simulink model "Q8"  (R2023a)
settings: Solver=VariableStepAuto  StartTime=0.0  StopTime=3  RelTol=1e-3
libraries: spsControlledVoltageSourceLib x3, spsAsynchronousMachineSIUnitsLib x1, spsGroundLib x1, eeProgrammableSignalGenerator x1, spspowerguiLib x1
settings Model: Creator=mango  LastModifiedBy=eij22jb
settings OptimizationCC: ReuseModelBlockBuffer=off

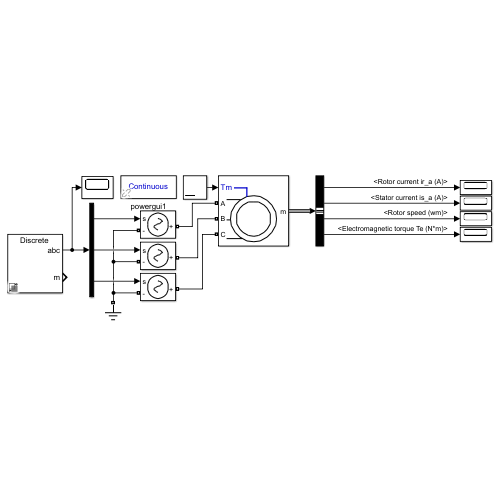
[thumbnail: Simulink's stored preview of the top-level diagram]
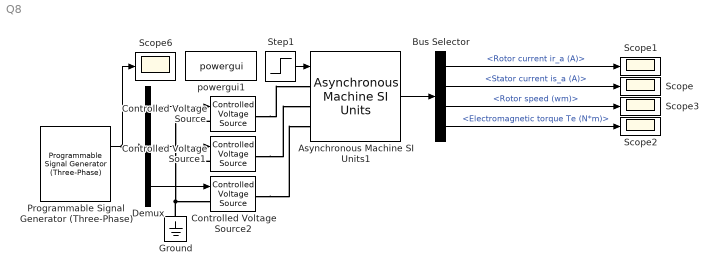
== system Q8 ==
  Asynchronous Machine SI Units1 : spsAsynchronousMachineSIUnitsLib/Asynchronous Machine SI Units  RotorType=Squirrel-cage  PresetModel=No  MechanicalLoad=Torque Tm  ShowDetailedParameters=on  ReferenceFrame=Rotor  Units=SI  MeasurementBus=off  NominalParameters=[9325 400 50]  VoltageRatio=1  Stator=[0.8 0.00907]  Rotor=[0.8 0.00907]  Cage1=[0.4155 0.002066]  Cage2=[0.4168 0.0003495]  Lm=0.637  Mechanical=[0.1 0 2]  PolePairs=2  InitialConditions=[1 0 0 0 0 0 0 0]  SimulateSaturation=off  Saturation=[14.03593122, 27.81365428, 53.79336849, 72.68890987, 97.98006896, 148.6815601, 215.7428561, 302.9841135, 428.7778367 ; 230, 322, 414, 460, 506, 552, 598, 644, 690]  LoadFlowParameters=1492000  TsPowergui=0  TsBlock=-1  IterativeModel=Trapezoidal non iterative  IterativeDiscreteModel=Trapezoidal non iterative  Pmec=1.492e+006
  Bus Selector : BusSelector  OutputSignals=Rotor measurements.Rotor current ir_a (A),Stator measurements.Stator current is_a (A),Mechanical.Rotor speed (wm),Mechanical.Electromagnetic torque Te (N*m)
  Controlled Voltage Source : spsControlledVoltageSourceLib/Controlled Voltage Source  Initialize=on  Source_Type=AC  Amplitude=0  Phase=0  Frequency=0  Measurements=None
  Controlled Voltage Source1 : spsControlledVoltageSourceLib/Controlled Voltage Source  Initialize=on  Source_Type=AC  Amplitude=0  Phase=-120  Frequency=0  Measurements=None
  Controlled Voltage Source2 : spsControlledVoltageSourceLib/Controlled Voltage Source  Initialize=on  Source_Type=AC  Amplitude=0  Phase=0  Frequency=0  Measurements=None
  Demux : Demux  Outputs=3
  Ground : spsGroundLib/Ground  LConnTagsString=a
  Programmable Signal Generator (Three-Phase) : eeProgrammableSignalGenerator/Programmable Signal Generator (Three-Phase)  LabelModeActiveChoice=Discrete  VariationAmplitude=Ramp  Amp=0  Amp_RampRate=230*sqrt(2)/0.5  Amp_StepValue=100  Amp_ModulationMag=50  Amp_ModulationFreq=10  Amp_Tstart=0  Amp_Tstop=0.5  Amp_Table=[0 30 60 90]  Amp_Time=[0 0.3 0.6 0.9]  VariationFrequency=Ramp  Freq=5  Freq_RampRate=45/0.5  Freq_StepValue=100  Freq_ModulationMag=50  Freq_ModulationFreq=10  Freq_Tstart=0  Freq_Tstop=0.5  Freq_Table=[0 30 60 90]  Freq_Time=[0 0.3 0.6 0.9]  VariationPhase=Constant  Phase=0  Phase_RampRate=100  Phase_StepValue=100  Phase_ModulationMag=50  Phase_ModulationFreq=10  Phase_Tstart=0.1  Phase_Tstop=0.6  Phase_Table=[0 30 60 90]  Phase_Time=[0 0.3 0.6 0.9]  Harmo_En1=off  Harmo_Seq1=Zero Sequence  Harmo_Ord1=3  Harmo_Mag1=50  Harmo_Phase1=180  Harmo_Tstart1=0.1  Harmo_Tstop1=0.6  Harmo_En2=off  Harmo_Seq2=Zero Sequence  Harmo_Ord2=3  Harmo_Mag2=50  Harmo_Phase2=180  Harmo_Tstart2=0.1  Harmo_Tstop2=0.6  Ts=1e-4
      settings: LibrarySourceBlock=|
      | ee_sl_lib/General Control/Programmable
      | Signal Generator (Three-Phase)
  Scope{,1..3,6} (5 alike) : Scope
  Step1 : Step  Time=1.5  After=49.89  SampleTime=0
  powergui1 : spspowerguiLib/powergui  Priority=1  SimulationMode=Continuous  SampleTime=50e-6  frequency=60  Iterations=50  frequencyindice=50  Pbase=100e6  ErrMax=1e-4  UnitsV=kV  UnitsW=MW  buscounter=0  FunctionMessages=off  echomessages=off  EnableUseOfTLC=off  CurrentSourceSwitches=off  DisableSnubberDevices=off  DisableRonSwitches=off  DisableVfSwitches=off  DisplayEquations=off  AutomaticDiscreteSolvers=off  SolverType=Tustin/Backward Euler (TBE)  Interpol=off  ExternalGateDelay=off  methode=off  Ts=100  x0status=blocks  SPID=on  SwTol=0  HookPort=off  NonlinearTolerance=1e-4  nMaxIteration=100  ContinueOnMaxIteration=off  RestoreLinks=warning  ResistiveCurrentMeasurement=off  Frange=[0:2:500]  Ylog=off  Xlog=on  ShowGrid=off  save=off  variable=ZData  structure=0  ZoomFFT=off  StartTime=0.0  cycles=1  DisplayStyle=1  fundamental=60  FreqAxis=off  MaxFrequency=1000  frequencyindicesteady=1  RmsSteady=1  display=off
  wires:
  Asynchronous Machine SI Units1/1 -> Bus Selector/1
  Bus Selector/3 -> Scope3/1  "<Rotor speed (wm)>"
  Bus Selector/1 -> Scope1/1  "<Rotor current ir_a (A)>"
  Bus Selector/2 -> Scope/1  "<Stator current is_a (A)>"
  Bus Selector/4 -> Scope2/1  "<Electromagnetic torque Te (N*m)>"
  Step1/1 -> Asynchronous Machine SI Units1/1
  Demux/1 -> Controlled Voltage Source/1
  Demux/2 -> Controlled Voltage Source1/1
  Demux/3 -> Controlled Voltage Source2/1
  Programmable Signal Generator (Three-Phase)/1 -> Scope6/1, Demux/1
  connections:
  Ground/LConn1 -- Controlled Voltage Source/LConn1 -- Controlled Voltage Source1/LConn1 -- Controlled Voltage Source2/LConn1
  Controlled Voltage Source/RConn1 -- Asynchronous Machine SI Units1/LConn1
  Controlled Voltage Source1/RConn1 -- Asynchronous Machine SI Units1/LConn2
  Controlled Voltage Source2/RConn1 -- Asynchronous Machine SI Units1/LConn3
